simulink model "LB_PathTracAdptVel_EKF"  (Simulink 9.2)
settings: Solver=ode4  StartTime=0  StopTime=400  FixedStep=1e-3  RelTol=1e-6  AbsTol=1e-6
InitFcn:
  | clear;
  | close all
StopFcn:
  | close all;
  | t=tout(1:length(Vel_Trg));
  | figure
  | subplot(2,1,1)
  | plot(PreView_X,PreView_Y,'r','LineWidth',1.5);
  | hold on
  | plot(Current_Position(:,1),Current_Position(:,2),'k','LineWidth',1.5);
  | legend('Preview Position','Current Position');
  | 
  | subplot(2,1,2)
  | plot(Cur_Yaw,'r','LineWidth',1.5);
  | hold on
  | plot(PreViewHeading,'k','LineWidth',1.5);
  | legend('Current Heading','PreView Heading');
  | 
  | figure
  | subplot(3,1,1)
  | plot(Delta_Lateral,'k','LineWidth',1.5);
  | legend('Lateral Errors');
  | subplot(3,1,2)
  | plot(Heading_error,'r','LineWidth',1.5);
  | legend('Heading  Errors');
  | subplot(3,1,3)
  | plot(SteerCmd,'k','LineWidth',1.5);
  | legend('Steering Command');
  | 
  | % figure
  | % subplot(2,1,1)
  | % plot(ax_Cur,'k','LineWidth',1.5);
  | % legend('Longitudinal Acceleration')
  | % hold on
  | % subplot(2,1,2)
  | % plot(ay_Cur,'r','LineWidth',1.5);
  | % legend('Lateral Acceleration')
  | 
  | %% 加噪后的测量vs真实值
  | figure1=figure;
  | axes1 = axes('Parent',figure1);
  | hold(axes1,'on');
  | plot(Xo_Ce,Yo_Ce,'b','LineWidth',1)
  | hold on
  | plot(Xo_Cur,Yo_Cur,'-.r','LineWidth',2)
  | legend('测量值','真实值')
  | % 创建 ylabel
  | ylabel({'Y-m'});
  | xlabel({'X-m'});
  | box(axes1,'on');
  | grid(axes1,'on');
  | % 设置其余坐标区属性
  | set(axes1,'FontName','Times New Roman','FontWeight','bold');
  | 
  | 
  | figure2=figure;
  | axes2 = axes('Parent',figure2);
  | hold(axes2,'on');
  | plot(t,ax_Ce,'b','LineWidth',1)
  | hold on
  | plot(t,ax_Cur,'-.r','LineWidth',2)
  | legend('测量值','真实值')
  | % 创建 ylabel
  | ylabel({'纵向加速度-m/s^2'});
  | xlabel({'时间-s'});
  | box(axes2,'on');
  | grid(axes2,'on');
  | % 设置其余坐标区属性
  | set(axes2,'FontName','Times New Roman','FontWeight','bold');
  | 
  | figure4=figure;
  | axes4 = axes('Parent',figure4);
  | hold(axes4,'on');
  | plot(t,ay_Ce,'b','LineWidth',1)
  | hold on
  | plot(t,ay_Cur,'-.r','LineWidth',2)
  | legend('测量值','真实值')
  | % 创建 ylabel
  | ylabel({'横向加速度-m/s^2'});
  | xlabel({'时间-s'});
  | box(axes4,'on');
  | grid(axes4,'on');
  | % 设置其余坐标区属性
  | set(axes4,'FontName','Times New Roman','FontWeight','bold');
  | 
  | figure3=figure;
  | axes3 = axes('Parent',figure3);
  | hold(axes3,'on');
  | plot(t,Yaw_Ce,'b','LineWidth',1)
  | hold on
  | plot(t,Yaw_Cur,'-.r','LineWidth',2)
  | legend('测量值','真实值')
  | % 创建 ylabel
  | ylabel({'横摆角-rad'});
  | xlabel({'时间-s'});
  | box(axes3,'on');
  | grid(axes3,'on');
  | % 设置其余坐标区属性
  | set(axes3,'FontName','Times New Roman','FontWeight','bold');
  | %% EKF 结果图
  | figure_Position=figure;
  | axes4 = axes('Parent',figure_Position);
  | hold(axes4,'on');
  | plot(X_Groud_Truth(:,1),X_Groud_Truth(:,2),'r','LineWidth',2)
  | hold on
  | % plot(tout,Yaw,'-.r','LineWidth',2)
  | plot(X_EKF_Opt(:,1),X_EKF_Opt(:,2),'b','LineWidth',2)
  | plot(X_Ce_Current(:,1),X_Ce_Current(:,2),'k','LineWidth',2)
  | legend('真实值','EKF-估计','测量值')
  | % 创建 ylabel
  | ylabel({'Y-m'});
  | xlabel({'X-m'});
  | box(axes4,'on');
  | grid(axes4,'on');
  | % 设置其余坐标区属性
  | set(axes4,'FontName','Times New Roman','FontWeight','bold');
  | 
  | figure_Yaw=figure;
  | axes5 = axes('Parent',figure_Yaw);
  | hold(axes5,'on');
  | plot(t,X_Groud_Truth(:,3),'r','LineWidth',2)
  | hold on
  | plot(t,X_EKF_Opt(:,3),'b','LineWidth',2)
  | plot(t,X_Ce_Current(:,3),'k','LineWidth',2)
  | legend('真实值','EKF-估计','测量值')
  | % 创建 ylabel
  | ylabel({'航向角-rad'});
  | xlabel({'时间-s'});
  | box(axes5,'on');
  | grid(axes5,'on');
  | % 设置其余坐标区属性
  | set(axes5,'FontName','Times New Roman','FontWeight','bold');
  | 
  | figure_YawRate=figure;
  | axes6 = axes('Parent',figure_YawRate);
  | hold(axes6,'on');
  | plot(t,X_Groud_Truth(:,4),'r','LineWidth',2)
  | hold on
  | plot(t,X_EKF_Opt(:,4),'b','LineWidth',2)
  | plot(t,X_Ce_Current(:,4),'k','LineWidth',2)
  | legend('真实值','EKF-估计','测量值')
  | % 创建 ylabel
  | ylabel({'横摆角速度-rad/s'});
  | xlabel({'时间-s'});
  | box(axes6,'on');
  | grid(axes6,'on');
  | % 设置其余坐标区属性
  | set(axes6,'FontName','Times New Roman','FontWeight','bold');
  | 
  | figure_Vx=figure;
  | axes7 = axes('Parent',figure_Vx);
  | hold(axes7,'on');
  | plot(t,X_Groud_Truth(:,5),'r','LineWidth',2)
  | hold on
  | plot(t,X_EKF_Opt(:,5),'b','LineWidth',2)
  | % plot(t,X_Ce_Current(:,4),'k','LineWidth',2)
  | legend('真实值','EKF-估计')
  | % 创建 ylabel
  | ylabel({'纵向车速-m/s'});
  | xlabel({'时间-s'});
  | box(axes7,'on');
  | grid(axes7,'on');
  | % 设置其余坐标区属性
  | set(axes7,'FontName','Times New Roman','FontWeight','bold');
  | 
  | figure_Vy=figure;
  | axes8 = axes('Parent',figure_Vy);
  | hold(axes8,'on');
  | plot(t,X_Groud_Truth(:,6),'r','LineWidth',2)
  | hold on
  | plot(t,X_EKF_Opt(:,6),'b','LineWidth',2)
  | % plot(t,X_Ce_Current(:,4),'k','LineWidth',2)
  | legend('真实值','EKF-估计')
  | % 创建 ylabel
  | ylabel({'横向车速-m/s'});
  | xlabel({'时间-s'});
  | box(axes8,'on');
  | grid(axes8,'on');
  | % 设置其余坐标区属性
  | set(axes8,'FontName','Times New Roman','FontWeight','bold');
libraries: simulink x9, Solver_SF x1
settings Model: Creator=ywata  LastModifiedBy=Administrator  SimulationMode=accelerator  ExtModeTrigMode=oneshot  ExtModeArmWhenConnect=off
settings SolverCC: AutoScaleAbsTol=off
settings DataIOCC: LimitDataPoints=off  SignalLoggingName=sigsOut
settings OptimizationCC: BlockReduction=off  BooleanDataType=off
settings DebuggingCC: SaveWithParameterizedLinksMsg=none  SignalResolutionControl=TryResolveAllWithWarning  MultiTaskDSMMsg=warning  MultiTaskCondExecSysMsg=none
settings HardwareCC: TargetUnknown=on
settings RTWCC: TemplateMakefile=grt_vc.tmf
settings GRTTargetCC: TargetFcnLib=ansi_tfl_tmw.mat

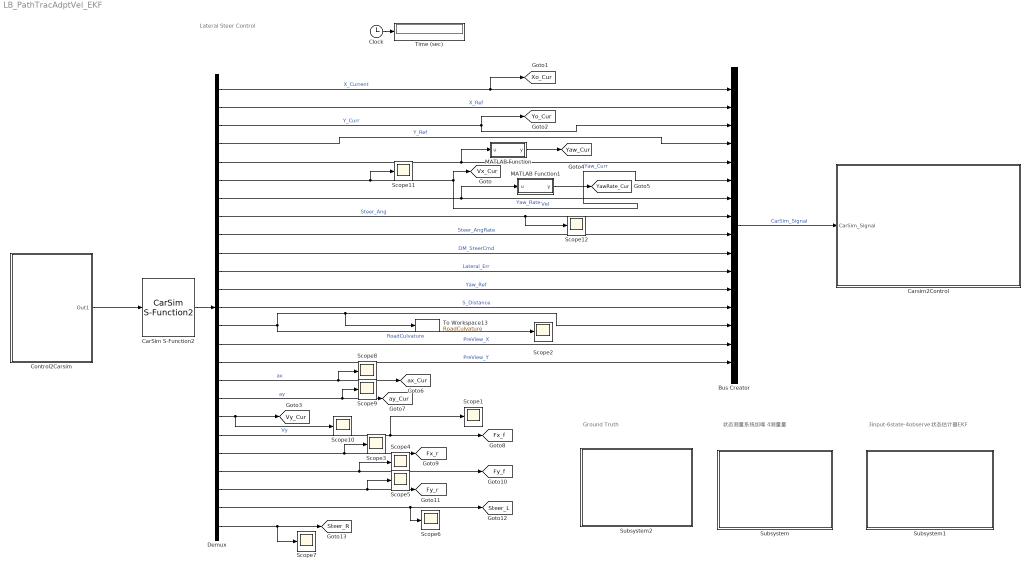
== system LB_PathTracAdptVel_EKF ==
  note: Lateral Steer Control
  note: 状态测量系统加噪
      | 4测量量
  note: 3input-6state-4observe状态估计器EKF
  note: Ground Truth
  Bus Creator : BusCreator  Inputs=16
  CarSim S-Function2 : Solver_SF/CarSim S-Function2  Priority=1  VehicleCode=i_i  SIMFILE=simfile.sim
      settings: AttributesFormatString=Vehicle Code: %<VehicleCode>
  Carsim2Control : Subsystem
  Clock : Clock
  Control2Carsim : Subsystem
  Demux : Demux  Outputs=25
  MATLAB Function : MATLAB Function  TreatAsAtomicUnit=on
  MATLAB Function1 : MATLAB Function  TreatAsAtomicUnit=on
  Scope{1..12} (12 alike) : Scope
  Subsystem : Subsystem
  Subsystem1 : Subsystem
  Subsystem2 : Subsystem
  Time (sec) : Display
      settings: Format=bank  Decimation=100
  To Workspace13 : ToWorkspace  VariableName=RoadCulvature  SampleTime=-1
  tag scope: Fx_f=global, Fx_r=global, Fy_f=global, Fy_r=global, Steer_L=global, Steer_R=global, Vx_Cur=global, Vy_Cur=global, Xo_Cur=global, YawRate_Cur=global, Yaw_Cur=global, Yo_Cur=global, ax_Cur=global, ay_Cur=global
  wires:
  CarSim S-Function2/1 -> Demux/1
  Clock/1 -> Time (sec)/1
  Demux/1 -> [Xo_Cur], Bus Creator/1  "X_Current"
  Demux/2 -> Bus Creator/2  "X_Ref"
  Demux/3 -> [Yo_Cur], Bus Creator/3  "Y_Curr"
  Demux/4 -> Bus Creator/4  "Y_Ref"
  Demux/5 -> MATLAB Function/1(u), Bus Creator/5  "Yaw_Curr"
  Demux/6 -> Scope11/1, [Vx_Cur], Bus Creator/6  "Vel"
  Demux/8 -> Scope12/1, Bus Creator/8  "Steer_Ang"
  Demux/9 -> Bus Creator/9  "Steer_AngRate"
  Demux/10 -> Bus Creator/10  "DM_SteerCmd"
  Demux/11 -> Bus Creator/11  "Lateral_Err"
  Demux/12 -> Bus Creator/12  "Yaw_Ref"
  Demux/13 -> Bus Creator/13  "S_Distance"
  Demux/14 -> Scope2/1, To Workspace13/1, Bus Creator/14  "RoadCulvature"
  Demux/15 -> Bus Creator/15  "PreView_X"
  Demux/16 -> Bus Creator/16  "PreView_Y"
  Bus Creator/1 -> Carsim2Control/1(CarSim_Signal)  "CarSim_Signal"
  Control2Carsim/1(Out1) -> CarSim S-Function2/1
  Demux/18 -> Scope9/1, [ay_Cur]  "ay"
  Demux/17 -> Scope8/1, [ax_Cur]  "ax"
  MATLAB Function1/1(y) -> [YawRate_Cur]
  Demux/7 -> MATLAB Function1/1(u), Bus Creator/7  "Yaw_Rate"
  MATLAB Function/1(y) -> [Yaw_Cur]
  Demux/19 -> Scope10/1, [Vy_Cur]  "Vy"
  Demux/20 -> Scope1/1, [Fx_f]
  Demux/21 -> Scope3/1, [Fx_r]
  Demux/22 -> Scope4/1, [Fy_f]
  Demux/23 -> Scope5/1, [Fy_r]
  Demux/24 -> Scope6/1, [Steer_L]
  Demux/25 -> Scope7/1, [Steer_R]

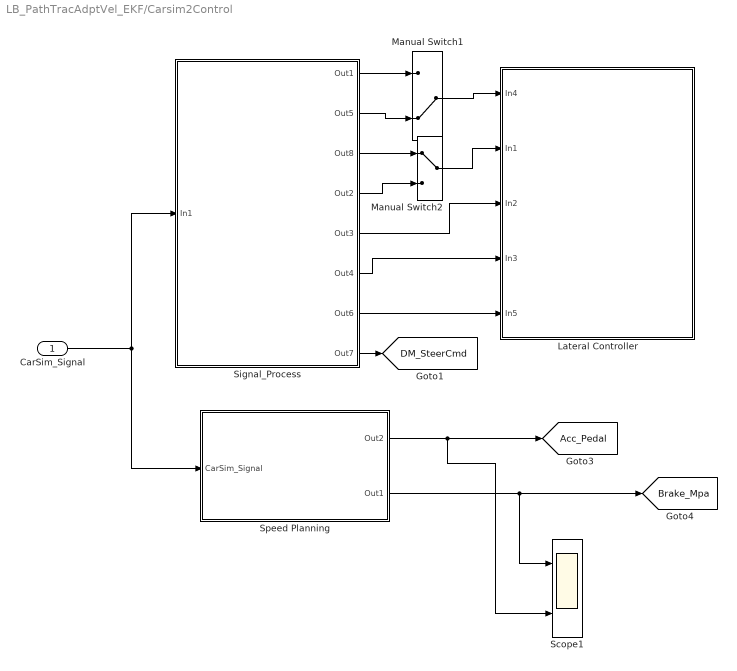
== system LB_PathTracAdptVel_EKF/Carsim2Control ==
  CarSim_Signal : Inport
  Lateral Controller : Subsystem
  Manual Switch1 : ManualSwitch  CurrentSetting=0
  Manual Switch2 : ManualSwitch
  Scope1 : Scope  NumInputPorts=2
  "Signal_Process " : Subsystem
  Speed Planning : Subsystem
  tag scope: Acc_Pedal=global, Brake_Mpa=global, DM_SteerCmd=global
  wires:
  "Signal_Process "/7(Out6) -> Lateral Controller/5(In5)
  Manual Switch1/1 -> Lateral Controller/1(In4)
  CarSim_Signal/1 -> Speed Planning/1(CarSim_Signal), "Signal_Process "/1(In1)
  "Signal_Process "/4(Out2) -> Manual Switch2/2
  Manual Switch2/1 -> Lateral Controller/2(In1)
  "Signal_Process "/2(Out5) -> Manual Switch1/2
  "Signal_Process "/8(Out7) -> [DM_SteerCmd]
  Speed Planning/1(Out2) -> Scope1/2, [Acc_Pedal]
  "Signal_Process "/3(Out8) -> Manual Switch2/1
  Speed Planning/2(Out1) -> Scope1/1, [Brake_Mpa]
  "Signal_Process "/1(Out1) -> Manual Switch1/1
  "Signal_Process "/5(Out3) -> Lateral Controller/3(In2)
  "Signal_Process "/6(Out4) -> Lateral Controller/4(In3)

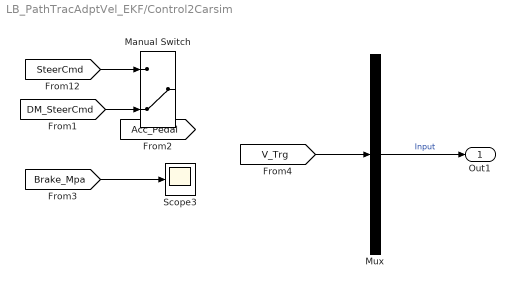
== system LB_PathTracAdptVel_EKF/Control2Carsim ==
  Manual Switch : ManualSwitch  CurrentSetting=0
  Mux : Mux  Inputs=1
  Scope3 : Scope
  Out1 : Outport
  wires:
  [SteerCmd] -> Manual Switch/1
  Mux/1 -> Out1/1  "Input"
  [DM_SteerCmd] -> Manual Switch/2
  [Brake_Mpa] -> Scope3/1
  [V_Trg] -> Mux/1

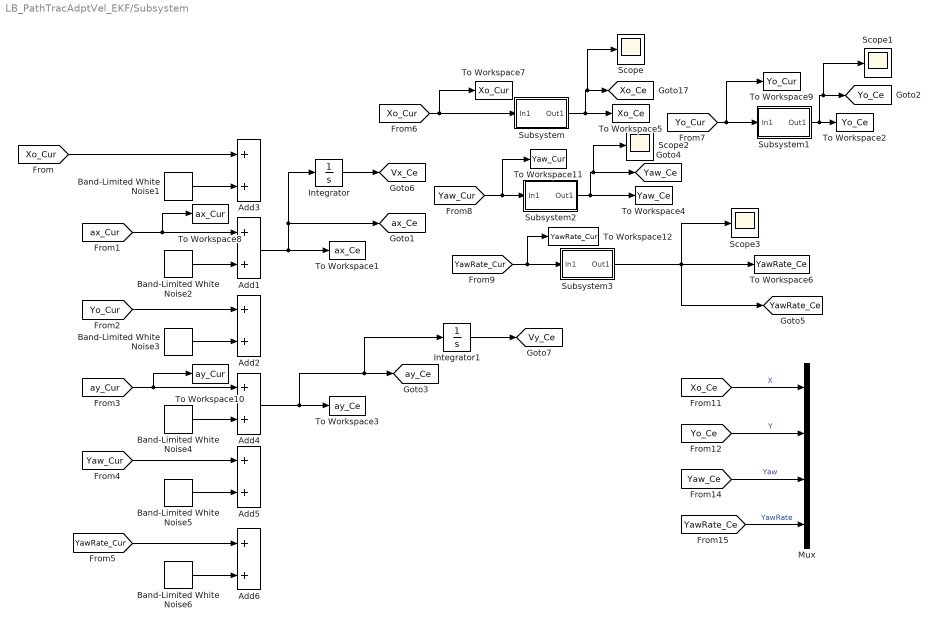
== system LB_PathTracAdptVel_EKF/Subsystem ==
  Add{1..6} (6 alike) : Sum
  Band-Limited White Noise1 : simulink/Sources/Band-Limited White Noise  Cov=0.0001*[0.1]  Ts=1e-3  seed=[23341]
  Band-Limited White Noise2 : simulink/Sources/Band-Limited White Noise  Cov=0.001*[0.1]  Ts=1e-3  seed=[23341]
  Band-Limited White Noise3 : simulink/Sources/Band-Limited White Noise  Cov=0.0001*[0.1]  Ts=1e-3  seed=[23341]
  Band-Limited White Noise4 : simulink/Sources/Band-Limited White Noise  Cov=0.001*[0.1]  Ts=1e-3  seed=[23341]
  Band-Limited White Noise5 : simulink/Sources/Band-Limited White Noise  Cov=0.000003*[0.1]  Ts=1e-3  seed=[23341]
  Band-Limited White Noise6 : simulink/Sources/Band-Limited White Noise  Cov=0.00003*[0.1]  Ts=1e-3  seed=[23341]
  Integrator : Integrator
  Integrator1 : Integrator
  Mux : Mux
  Scope{,1..3} (4 alike) : Scope
  Subsystem : Subsystem  mask{Delta=0.1}
      mask prompts: Delta "标准差"
  Subsystem1 : Subsystem  mask{Delta=0.1}
      mask prompts: Delta "标准差"
  Subsystem2 : Subsystem  mask{Delta=deg2rad(3)}
      mask prompts: Delta "标准差"
  Subsystem3 : Subsystem  mask{Delta=deg2rad(1)}
      mask prompts: Delta "标准差"
  To Workspace1 : ToWorkspace  VariableName=ax_Ce  SampleTime=-1
  To Workspace10 : ToWorkspace  VariableName=ay_Cur  SampleTime=-1
  To Workspace11 : ToWorkspace  VariableName=Yaw_Cur  SampleTime=-1
  To Workspace12 : ToWorkspace  VariableName=YawRate_Cur  SampleTime=-1
  To Workspace2 : ToWorkspace  VariableName=Yo_Ce  SampleTime=-1
  To Workspace3 : ToWorkspace  VariableName=ay_Ce  SampleTime=-1
  To Workspace4 : ToWorkspace  VariableName=Yaw_Ce  SampleTime=-1
  To Workspace5 : ToWorkspace  VariableName=Xo_Ce  SampleTime=-1
  To Workspace6 : ToWorkspace  VariableName=YawRate_Ce  SampleTime=-1
  To Workspace7 : ToWorkspace  VariableName=Xo_Cur  SampleTime=-1
  To Workspace8 : ToWorkspace  VariableName=ax_Cur  SampleTime=-1
  To Workspace9 : ToWorkspace  VariableName=Yo_Cur  SampleTime=-1
  tag scope: Vx_Ce=global, Vy_Ce=global, Xo_Ce=global, YawRate_Ce=global, Yaw_Ce=global, Yo_Ce=global, ax_Ce=global, ay_Ce=global
  wires:
  Band-Limited White Noise1/1 -> Add3/2
  [Xo_Cur] -> Add3/1
  [ax_Cur] -> To Workspace8/1, Add1/1
  Band-Limited White Noise2/1 -> Add1/2
  Band-Limited White Noise3/1 -> Add2/2
  [Yo_Cur] -> Add2/1
  [ay_Cur] -> To Workspace10/1, Add4/1
  Band-Limited White Noise4/1 -> Add4/2
  Add4/1 -> Integrator1/1, [ay_Ce], To Workspace3/1
  Band-Limited White Noise5/1 -> Add5/2
  [Yaw_Cur] -> Add5/1
  [YawRate_Cur] -> Add6/1
  Band-Limited White Noise6/1 -> Add6/2
  Add1/1 -> [ax_Ce], Integrator/1, To Workspace1/1
  Integrator/1 -> [Vx_Ce]
  Integrator1/1 -> [Vy_Ce]
  [Yaw_Ce] -> Mux/3  "Yaw"
  [YawRate_Ce] -> Mux/4  "YawRate"
  [Xo_Ce] -> Mux/1  "X"
  [Yo_Ce] -> Mux/2  "Y"
  Subsystem/1(Out1) -> Scope/1, [Xo_Ce], To Workspace5/1
  [Xo_Cur] -> To Workspace7/1, Subsystem/1(In1)
  [Yo_Cur] -> To Workspace9/1, Subsystem1/1(In1)
  Subsystem1/1(Out1) -> Scope1/1, [Yo_Ce], To Workspace2/1
  Subsystem2/1(Out1) -> To Workspace4/1, Scope2/1, [Yaw_Ce]
  [Yaw_Cur] -> To Workspace11/1, Subsystem2/1(In1)
  [YawRate_Cur] -> To Workspace12/1, Subsystem3/1(In1)
  Subsystem3/1(Out1) -> To Workspace6/1, Scope3/1, [YawRate_Ce]

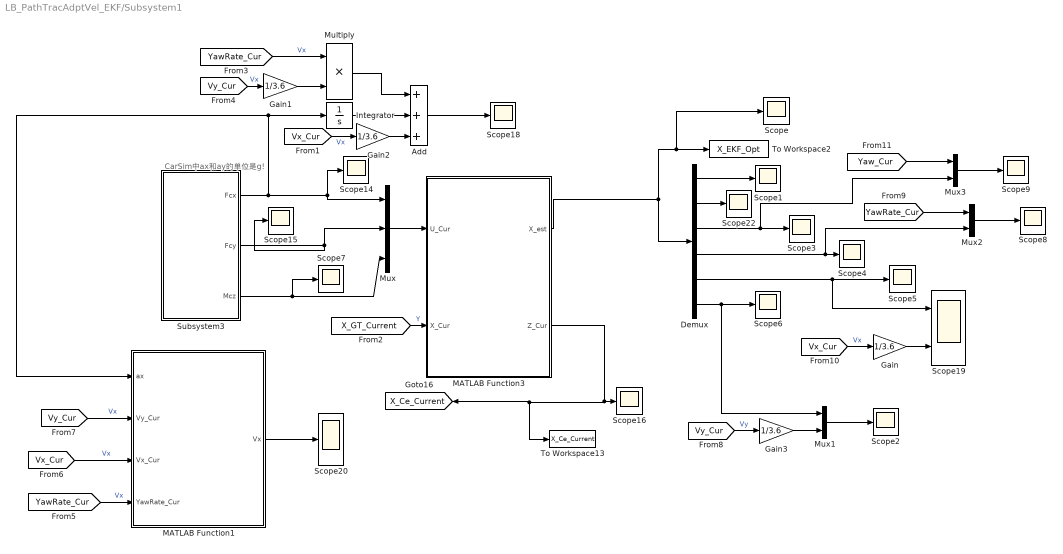
== system LB_PathTracAdptVel_EKF/Subsystem1 ==
  note: CarSim中ax和ay的单位是g!
  Add : Sum  Inputs=+++
  Demux : Demux  Outputs=6
  Gain{,1..3} (4 alike) : Gain  Gain=1/3.6
  Integrator : Integrator
  MATLAB Function1 : MATLAB Function  TreatAsAtomicUnit=on
  MATLAB Function3 : MATLAB Function  TreatAsAtomicUnit=on
  Multiply : Product
  Mux : Mux  Inputs=3
  Mux1 : Mux  Inputs=2
  Mux2 : Mux  Inputs=2
  Mux3 : Mux  Inputs=2
  Scope{,1..9,14..16,18,20,22} (16 alike) : Scope
  Scope19 : Scope  NumInputPorts=2
  Subsystem3 : Subsystem
  To Workspace13 : ToWorkspace  VariableName=X_Ce_Current  SampleTime=-1
      settings: Save2DSignal=2-D array (concatenate along first dimension)
  To Workspace2 : ToWorkspace  VariableName=X_EKF_Opt  SampleTime=-1
      settings: Save2DSignal=2-D array (concatenate along first dimension)
  tag scope: X_Ce_Current=global
  wires:
  [X_GT_Current] -> MATLAB Function3/2(X_Cur)  "Y"
  Demux/1 -> Scope1/1
  Demux/2 -> Scope22/1
  Demux/5 -> Scope19/1, Scope5/1
  Demux/6 -> Mux1/1, Scope6/1
  MATLAB Function3/1(X_est) -> Demux/1, Scope/1, To Workspace2/1
  MATLAB Function3/2(Z_Cur) -> To Workspace13/1, [X_Ce_Current], Scope16/1
  Mux/1 -> MATLAB Function3/1(U_Cur)
  Integrator/1 -> Add/2
  [Vx_Cur] -> Gain/1  "Vx"
  Gain/1 -> Scope19/2
  [Vx_Cur] -> Gain2/1  "Vx"
  Add/1 -> Scope18/1
  [YawRate_Cur] -> Multiply/1  "Vx"
  Gain1/1 -> Multiply/2
  [Vy_Cur] -> Gain1/1  "Vx"
  Multiply/1 -> Add/1
  Gain2/1 -> Add/3
  [YawRate_Cur] -> MATLAB Function1/4(YawRate_Cur)  "Vx"
  [Vx_Cur] -> MATLAB Function1/3(Vx_Cur)  "Vx"
  [Vy_Cur] -> MATLAB Function1/2(Vy_Cur)  "Vx"
  MATLAB Function1/1(Vx) -> Scope20/1
  Subsystem3/1(Fcx) -> Scope14/1, Mux/1, Integrator/1, MATLAB Function1/1(ax)
  Subsystem3/2(Fcy) -> Mux/2, Scope15/1
  Subsystem3/3(Mcz) -> Mux/3, Scope7/1
  [Vy_Cur] -> Gain3/1  "Vy"
  Gain3/1 -> Mux1/2
  Mux1/1 -> Scope2/1
  Mux2/1 -> Scope8/1
  Demux/4 -> Mux2/2, Scope4/1
  [YawRate_Cur] -> Mux2/1
  [Yaw_Cur] -> Mux3/1
  Demux/3 -> Mux3/2, Scope3/1
  Mux3/1 -> Scope9/1

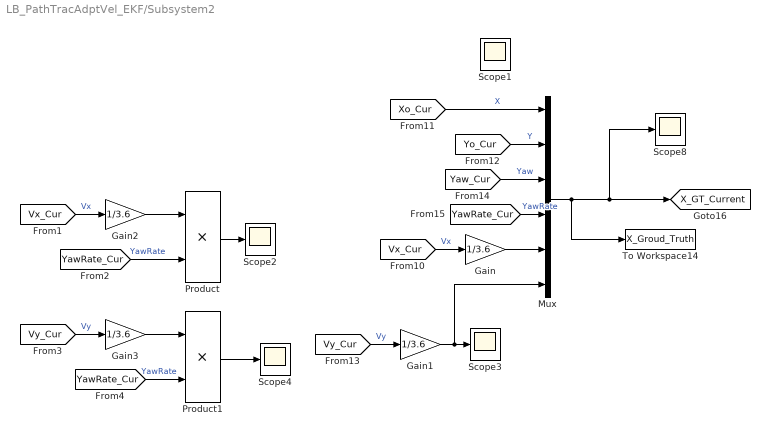
== system LB_PathTracAdptVel_EKF/Subsystem2 ==
  Gain{,1..3} (4 alike) : Gain  Gain=1/3.6
  Mux : Mux  Inputs=6
  Product : Product
  Product1 : Product
  Scope{1..4,8} (5 alike) : Scope
  To Workspace14 : ToWorkspace  VariableName=X_Groud_Truth  SampleTime=-1
      settings: Save2DSignal=2-D array (concatenate along first dimension)
  tag scope: X_GT_Current=global
  wires:
  [Xo_Cur] -> Mux/1  "X"
  Mux/1 -> To Workspace14/1, Scope8/1, [X_GT_Current]
  [Vy_Cur] -> Gain1/1  "Vy"
  [Vx_Cur] -> Gain/1  "Vx"
  Gain1/1 -> Mux/6, Scope3/1
  [Vx_Cur] -> Gain2/1  "Vx"
  Gain2/1 -> Product/1
  [YawRate_Cur] -> Product/2  "YawRate"
  Product/1 -> Scope2/1
  [Vy_Cur] -> Gain3/1  "Vy"
  Gain3/1 -> Product1/1
  [YawRate_Cur] -> Product1/2  "YawRate"
  Product1/1 -> Scope4/1
  [Yo_Cur] -> Mux/2  "Y"
  [Yaw_Cur] -> Mux/3  "Yaw"
  [YawRate_Cur] -> Mux/4  "YawRate"
  Gain/1 -> Mux/5

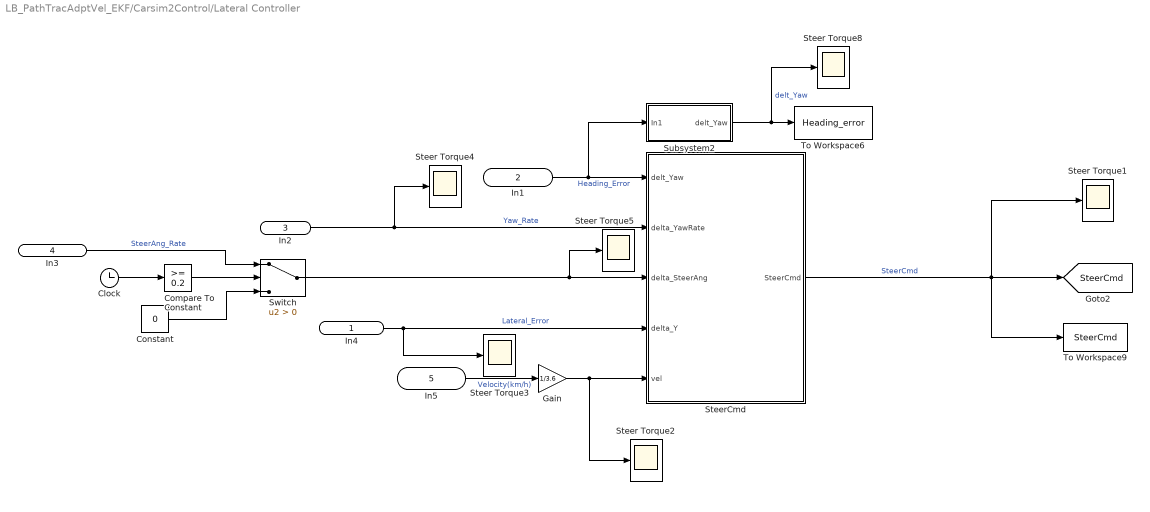
== system LB_PathTracAdptVel_EKF/Carsim2Control/Lateral Controller ==
  In4 : Inport
  In1 : Inport  Port=2
  In2 : Inport  Port=3
  In3 : Inport  Port=4
  In5 : Inport  Port=5
  Clock : Clock
  Compare To Constant : simulink/Logic and Bit Operations/Compare To Constant  relop=>=  const=0.2  OutDataTypeStr=boolean
  Constant : Constant  Value=0
  Gain : Gain  Gain=1/3.6
  Steer Torque{1..5,8} (6 alike) : Scope
  SteerCmd : MATLAB Function  TreatAsAtomicUnit=on
  Subsystem2 : Subsystem
  Switch : Switch  Criteria=u2 > Threshold
  To Workspace6 : ToWorkspace  VariableName=Heading_error  SampleTime=-1
  To Workspace9 : ToWorkspace  VariableName=SteerCmd  SampleTime=-1
  tag scope: SteerCmd=global
  wires:
  In5/1 -> Gain/1  "Velocity(km/h)"
  SteerCmd/1(SteerCmd) -> [SteerCmd], Steer Torque1/1, To Workspace9/1  "SteerCmd"
  Gain/1 -> Steer Torque2/1, SteerCmd/5(vel)
  In2/1 -> Steer Torque4/1, SteerCmd/2(delta_YawRate)  "Yaw_Rate"
  In1/1 -> Subsystem2/1(In1), SteerCmd/1(delt_Yaw)  "Heading_Error"
  In4/1 -> Steer Torque3/1, SteerCmd/4(delta_Y)  "Lateral_Error"
  Subsystem2/1(delt_Yaw) -> Steer Torque8/1, To Workspace6/1  "delt_Yaw"
  Clock/1 -> Compare To Constant/1
  Compare To Constant/1 -> Switch/2
  In3/1 -> Switch/1  "SteerAng_Rate"
  Constant/1 -> Switch/3
  Switch/1 -> Steer Torque5/1, SteerCmd/3(delta_SteerAng)

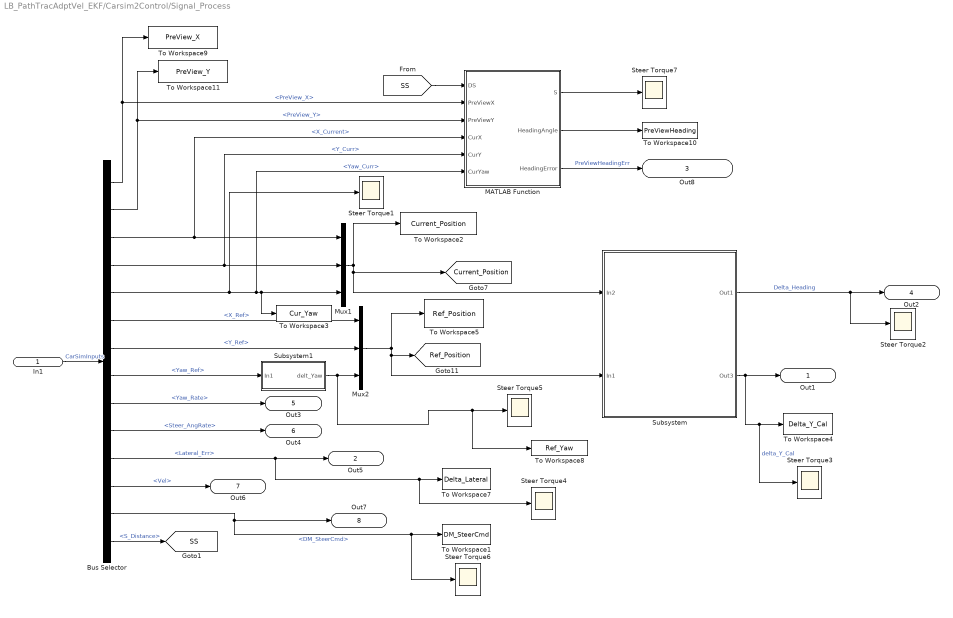
== system LB_PathTracAdptVel_EKF/Carsim2Control/Signal_Process  ==
  In1 : Inport
  Bus Selector : BusSelector  OutputSignals=PreView_X,PreView_Y,X_Current,Y_Curr,Yaw_Curr,X_Ref,Y_Ref,Yaw_Ref,Yaw_Rate,Steer_AngRate,Lateral_Err,Vel,DM_SteerCmd,S_Distance
  MATLAB Function : MATLAB Function  TreatAsAtomicUnit=on
  Mux1 : Mux  Inputs=3
  Mux2 : Mux  Inputs=3
  Steer Torque{1..7} (7 alike) : Scope
  Subsystem : Subsystem
  Subsystem1 : Subsystem
  To Workspace1 : ToWorkspace  VariableName=DM_SteerCmd  SampleTime=-1
  To Workspace10 : ToWorkspace  VariableName=PreViewHeading  SampleTime=-1
  To Workspace11 : ToWorkspace  VariableName=PreView_Y  SampleTime=-1
  To Workspace2 : ToWorkspace  VariableName=Current_Position  SampleTime=-1
  To Workspace3 : ToWorkspace  VariableName=Cur_Yaw  SampleTime=-1
  To Workspace4 : ToWorkspace  VariableName=Delta_Y_Cal  SampleTime=-1
  To Workspace5 : ToWorkspace  VariableName=Ref_Position  SampleTime=-1
  To Workspace7 : ToWorkspace  VariableName=Delta_Lateral  SampleTime=-1
  To Workspace8 : ToWorkspace  VariableName=Ref_Yaw  SampleTime=-1
  To Workspace9 : ToWorkspace  VariableName=PreView_X  SampleTime=-1
  Out1 : Outport
  Out5 : Outport  Port=2
  Out8 : Outport  Port=3
  Out2 : Outport  Port=4
  Out3 : Outport  Port=5
  Out4 : Outport  Port=6
  Out6 : Outport  Port=7
  Out7 : Outport  Port=8
  tag scope: Current_Position=global, Ref_Position=global, SS=global
  wires:
  Mux1/1 -> Subsystem/1(In2), [Current_Position], To Workspace2/1
  Bus Selector/6 -> Mux2/1  "<X_Ref>"
  Bus Selector/7 -> Mux2/2  "<Y_Ref>"
  Mux2/1 -> Subsystem/2(In1), [Ref_Position], To Workspace5/1
  Subsystem/1(Out1) -> Steer Torque2/1, Out2/1  "Delta_Heading"
  In1/1 -> Bus Selector/1  "CarSimInputs"
  Bus Selector/3 -> MATLAB Function/4(CurX), Mux1/1  "<X_Current>"
  Bus Selector/4 -> MATLAB Function/5(CurY), Mux1/2  "<Y_Curr>"
  Bus Selector/5 -> Steer Torque1/1, Mux1/3, To Workspace3/1, MATLAB Function/6(CurYaw)  "<Yaw_Curr>"
  Bus Selector/8 -> Subsystem1/1(In1)  "<Yaw_Ref>"
  Subsystem1/1(delt_Yaw) -> To Workspace8/1, Steer Torque5/1, Mux2/3
  Subsystem/2(Out3) -> Steer Torque3/1, To Workspace4/1, Out1/1  "delta_Y_Cal"
  Bus Selector/10 -> Out4/1  "<Steer_AngRate>"
  Bus Selector/9 -> Out3/1  "<Yaw_Rate>"
  Bus Selector/11 -> Steer Torque4/1, To Workspace7/1, Out5/1  "<Lateral_Err>"
  Bus Selector/12 -> Out6/1  "<Vel>"
  Bus Selector/13 -> Out7/1, Steer Torque6/1, To Workspace1/1  "<DM_SteerCmd>"
  Bus Selector/14 -> [SS]  "<S_Distance>"
  MATLAB Function/3(HeadingError) -> Out8/1  "PreViewHeadingErr"
  MATLAB Function/2(HeadingAngle) -> To Workspace10/1
  Bus Selector/1 -> To Workspace9/1, MATLAB Function/2(PreViewX)  "<PreView_X>"
  Bus Selector/2 -> To Workspace11/1, MATLAB Function/3(PreViewY)  "<PreView_Y>"
  MATLAB Function/1(S) -> Steer Torque7/1
  [SS] -> MATLAB Function/1(DS)

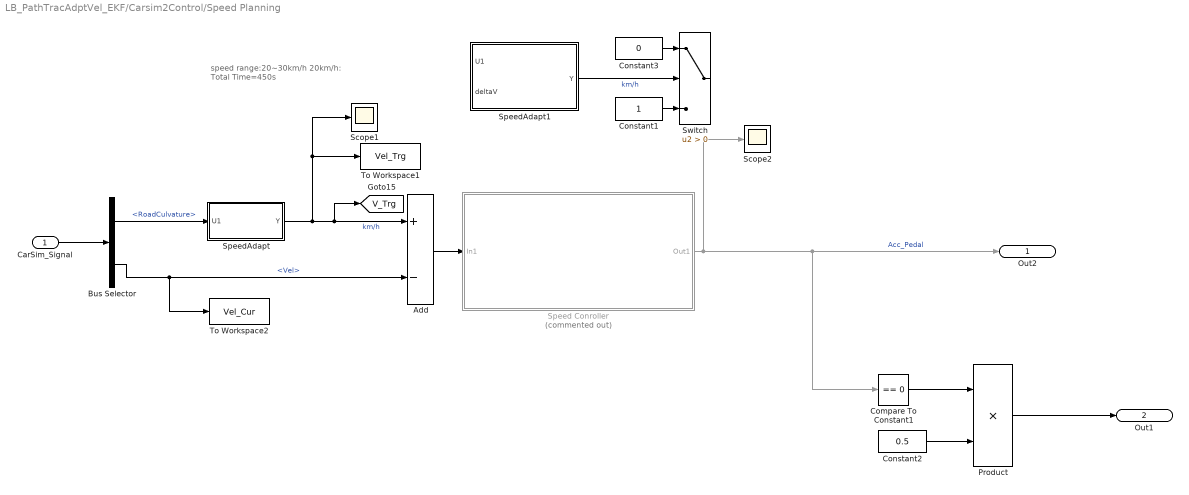
== system LB_PathTracAdptVel_EKF/Carsim2Control/Speed Planning ==
  note: speed range:20~30km/h
      | 20km/h: Total Time=450s
  CarSim_Signal : Inport
  Add : Sum  Inputs=+-
  Bus Selector : BusSelector  OutputSignals=RoadCulvature,Vel
  Compare To Constant1 : simulink/Logic and Bit Operations/Compare To Constant  relop===  const=0  OutDataTypeStr=boolean
  Constant1 : Constant
  Constant2 : Constant  Value=0.5
  Constant3 : Constant  Value=0
  Product : Product
  Scope1 : Scope
  Scope2 : Scope
  Speed Conroller : Subsystem  Commented=on
  SpeedAdapt : MATLAB Function  TreatAsAtomicUnit=on
  SpeedAdapt1 : MATLAB Function  TreatAsAtomicUnit=on
  Switch : Switch  Criteria=u2 > Threshold
  To Workspace1 : ToWorkspace  VariableName=Vel_Trg  SampleTime=-1
      settings: Save2DSignal=2-D array (concatenate along first dimension)
  To Workspace2 : ToWorkspace  VariableName=Vel_Cur  SampleTime=-1
      settings: Save2DSignal=2-D array (concatenate along first dimension)
  Out2 : Outport
  Out1 : Outport  Port=2
  tag scope: V_Trg=global
  wires:
  Add/1 -> Speed Conroller/1(In1)
  CarSim_Signal/1 -> Bus Selector/1
  Bus Selector/2 -> To Workspace2/1, Add/2  "<Vel>"
  Bus Selector/1 -> SpeedAdapt/1(U1)  "<RoadCulvature>"
  SpeedAdapt/1(Y) -> To Workspace1/1, Scope1/1, [V_Trg], Add/1  "km/h"
  Constant2/1 -> Product/2
  Speed Conroller/1(Out1) -> Out2/1, Compare To Constant1/1, Scope2/1  "Acc_Pedal"
  Constant1/1 -> Switch/3
  Constant3/1 -> Switch/1
  SpeedAdapt1/1(Y) -> Switch/2  "km/h"
  Compare To Constant1/1 -> Product/1
  Product/1 -> Out1/1

== system LB_PathTracAdptVel_EKF/Subsystem/Subsystem ==
  In1 : Inport
  Constant : Constant  Value=Delta
  MATLAB Function : MATLAB Function  TreatAsAtomicUnit=on
  Out1 : Outport
  wires:
  Constant/1 -> MATLAB Function/1(delta)
  In1/1 -> MATLAB Function/2(u)
  MATLAB Function/1(y) -> Out1/1

== system LB_PathTracAdptVel_EKF/Subsystem/Subsystem1 ==
  In1 : Inport
  Constant : Constant  Value=Delta
  MATLAB Function : MATLAB Function  TreatAsAtomicUnit=on
  Out1 : Outport
  wires:
  MATLAB Function/1(y) -> Out1/1
  In1/1 -> MATLAB Function/2(u)
  Constant/1 -> MATLAB Function/1(delta)

== system LB_PathTracAdptVel_EKF/Subsystem/Subsystem2 ==
  In1 : Inport
  Constant : Constant  Value=Delta
  MATLAB Function : MATLAB Function  TreatAsAtomicUnit=on
  Out1 : Outport
  wires:
  Constant/1 -> MATLAB Function/1(delta)
  In1/1 -> MATLAB Function/2(u)
  MATLAB Function/1(y) -> Out1/1

== system LB_PathTracAdptVel_EKF/Subsystem/Subsystem3 ==
  In1 : Inport
  Constant : Constant  Value=Delta
  MATLAB Function : MATLAB Function  TreatAsAtomicUnit=on
  Out1 : Outport
  wires:
  MATLAB Function/1(y) -> Out1/1
  In1/1 -> MATLAB Function/2(u)
  Constant/1 -> MATLAB Function/1(delta)

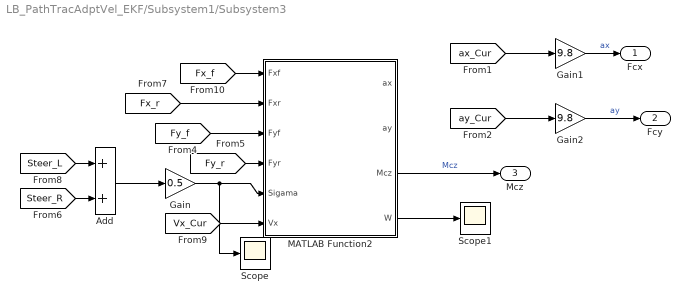
== system LB_PathTracAdptVel_EKF/Subsystem1/Subsystem3 ==
  Add : Sum
  Gain : Gain  Gain=0.5
  Gain1 : Gain  Gain=9.8
  Gain2 : Gain  Gain=9.8
  MATLAB Function2 : MATLAB Function  TreatAsAtomicUnit=on
  Scope : Scope
  Scope1 : Scope
  Fcx : Outport
  Fcy : Outport  Port=2
  Mcz : Outport  Port=3
  wires:
  [Fy_r] -> MATLAB Function2/4(Fyr)
  [Vx_Cur] -> MATLAB Function2/6(Vx)
  [Fy_f] -> MATLAB Function2/3(Fyf)
  MATLAB Function2/3(Mcz) -> Mcz/1  "Mcz"
  [ay_Cur] -> Gain2/1
  [ax_Cur] -> Gain1/1
  [Steer_L] -> Add/1
  [Steer_R] -> Add/2
  Add/1 -> Gain/1
  Gain/1 -> Scope/1, MATLAB Function2/5(Sigama)
  [Fx_r] -> MATLAB Function2/2(Fxr)
  [Fx_f] -> MATLAB Function2/1(Fxf)
  Gain1/1 -> Fcx/1  "ax"
  Gain2/1 -> Fcy/1  "ay"
  MATLAB Function2/4(W) -> Scope1/1

== system LB_PathTracAdptVel_EKF/Carsim2Control/Lateral Controller/Subsystem2 ==
  In1 : Inport
  Rad2Deg1 : MATLAB Function  TreatAsAtomicUnit=on
  delt_Yaw : Outport
  wires:
  Rad2Deg1/1(Y) -> delt_Yaw/1  "Deg"
  In1/1 -> Rad2Deg1/1(U1)  "rad"

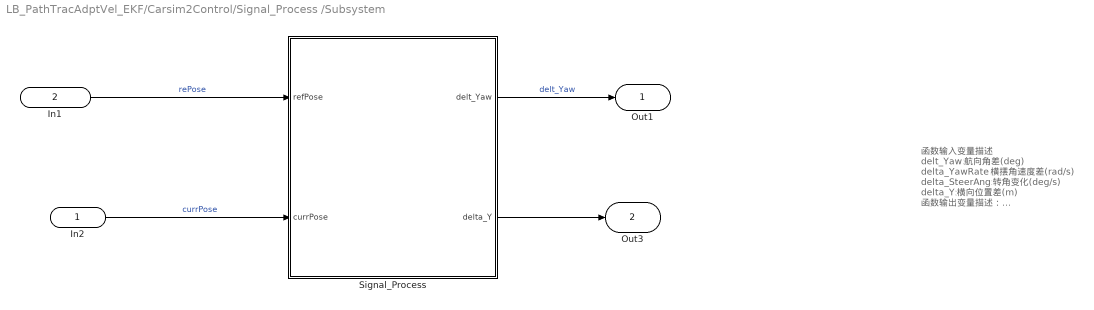
== system LB_PathTracAdptVel_EKF/Carsim2Control/Signal_Process /Subsystem ==
  note: 函数输入变量描述
      | delt_Yaw:航向角差(deg)
      | delta_YawRate:横摆角速度差(rad/s)
      | delta_SteerAng:转角变化(deg/s)
      | delta_Y:横向位置差(m)
      | 函数输出变量描述：
      | SteerCmd:前轮转角（degree）
  In2 : Inport
  In1 : Inport  Port=2
  Signal_Process : MATLAB Function  TreatAsAtomicUnit=on
  Out1 : Outport
  Out3 : Outport  Port=2
  wires:
  In1/1 -> Signal_Process/1(refPose)  "rePose"
  Signal_Process/1(delt_Yaw) -> Out1/1  "delt_Yaw"
  In2/1 -> Signal_Process/2(currPose)  "currPose"
  Signal_Process/2(delta_Y) -> Out3/1

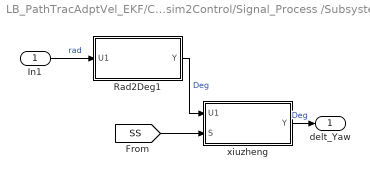
== system LB_PathTracAdptVel_EKF/Carsim2Control/Signal_Process /Subsystem1 ==
  In1 : Inport
  Rad2Deg1 : MATLAB Function  TreatAsAtomicUnit=on
  xiuzheng : MATLAB Function  TreatAsAtomicUnit=on
  delt_Yaw : Outport
  wires:
  In1/1 -> Rad2Deg1/1(U1)  "rad"
  Rad2Deg1/1(Y) -> xiuzheng/1(U1)  "Deg"
  [SS] -> xiuzheng/2(S)
  xiuzheng/1(Y) -> delt_Yaw/1  "Deg"

== system LB_PathTracAdptVel_EKF/Carsim2Control/Speed Planning/Speed Conroller ==
  In1 : Inport
  Constant : Constant  Value=0.2
  Constant1 : Constant  Value=0.1
  Discrete Varying PID : simulink/Continuous/PID Controller  Controller=PI  Form=Parallel  TimeDomain=Discrete-time  SampleTime=-1  IntegratorMethod=Forward Euler  FilterMethod=Forward Euler  ControllerParametersSource=external  P=1  I=1  D=0  UseFilter=on  N=100  TunerSelectOption=Transfer Function Based (PID Tuner App)  InitialConditionSource=internal  InitialConditionForIntegrator=0  InitialConditionForFilter=0  DifferentiatorICPrevScaledInput=0  ExternalReset=none  TrackingMode=off  Kt=1  LimitOutput=on  UpperSaturationLimit=1  LowerSaturationLimit=0  LinearizeAsGain=on  AntiWindupMode=none  Kb=1  POutMin=[]  POutMax=[]  IOutMin=[]  IOutMax=[]  DOutMin=[]  DOutMax=[]  NOutMin=[]  NOutMax=[]  SumOutMin=[]  SumOutMax=[]  SaturationOutMin=[]  SaturationOutMax=[]  PParamMin=[]  PParamMax=[]  IParamMin=[]  IParamMax=[]  DParamMin=[]  DParamMax=[]  NParamMin=[]  NParamMax=[]  KbParamMin=[]  KbParamMax=[]  KtParamMin=[]  KtParamMax=[]  KbOutMin=[]  KbOutMax=[]  KtOutMin=[]  KtOutMax=[]  IntegratorOutMin=[]  IntegratorOutMax=[]  FilterOutMin=[]  FilterOutMax=[]  SumI1OutMin=[]  SumI1OutMax=[]  SumI2OutMin=[]  SumI2OutMax=[]  SumI3OutMin=[]  SumI3OutMax=[]  SumI4OutMin=[]  SumI4OutMax=[]  SumDOutMin=[]  SumDOutMax=[]  DifferentiatorOutMin=[]  DifferentiatorOutMax=[]  FilterDiffOutCoefMin=[]  FilterDiffOutCoefMax=[]  ReciprocalOutMin=[]  ReciprocalOutMax=[]  SumDenOutMin=[]  SumDenOutMax=[]  SumNumOutMin=[]  SumNumOutMax=[]  DivideOutMin=[]  DivideOutMax=[]  IntegratorContinuousStateAttributes=''  IntegratorStateMustResolveToSignalObject=off  IntegratorRTWStateStorageClass=Auto  FilterContinuousStateAttributes=''  FilterStateMustResolveToSignalObject=off  FilterRTWStateStorageClass=Auto  ParallelPVariant=ExternalParameters  IdealPVariant=Disabled  IVariant=ExternalParameters  DVariant=Disabled  IntegratorVariant=Discrete  SatVariant=Enabled  AWVariant=Passthrough  PCopyVariant=Disabled  TRVariant=Disabled  FdbkBlocksVariant=Forward  IdealPFdbkVariant=Disabled  SatFdbkVariant=Disabled  DerivativeFilterVariant=Disabled  NVariant=Disabled  NCopyVariant=Disabled_SignalSpec  FilterICVariant=Disabled  IntegratorICVariant=InternalICs  ExternalResetVariant=Disabled  TRSumVariant=Passthrough  SumFdbkVariant=Disabled  SumVariant=Sum_PI
  Out1 : Outport
  wires:
  Constant/1 -> Discrete Varying PID/3
  In1/1 -> Discrete Varying PID/1  "Error_Spd"
  Constant1/1 -> Discrete Varying PID/2
  Discrete Varying PID/1 -> Out1/1  "Acc_Pedal"

== matlab function Carsim2Control/Signal_Process /Subsystem/Signal_Process ==
  data: refPose input double; delt_Yaw output double; currPose input double; delta_Y output double
function [delt_Yaw,delta_Y] = Signal_Process(refPose, currPose)
 % Clip heading angle to be within [0, 360) and convert to radian
refPose(3) = matlabshared.planning.internal.angleUtilities.convertAndWrapTo2Pi(refPose(3));
currPose(3)= matlabshared.planning.internal.angleUtilities.convertAndWrapTo2Pi(currPose(3));
delt_Yaw=matlabshared.planning.internal.angleUtilities.angdiff(refPose(3), currPose(3));
direction=1;
wheelbase=3;
delta_Y = computePositionError(refPose, currPose, direction, wheelbase);
end

 function delta_Y = computePositionError(refPose, currPose, direction, wheelbase)
% %computePositionError Compute the distance error
% 
% Tangent direction of the reference path
tHat = [cos(refPose(3)), sin(refPose(3))];

% Tracking error vector
if 1
    [poseF1,poseF2] = rearToFrontPose(currPose, wheelbase);
    d1 = poseF1 - refPose(1);
    d2 = poseF2 - refPose(2);

else
    d1 = currPose(1)  - refPose(1);
    d2 = currPose(2)  - refPose(2);
end
% 
% % Implement equation (8) in reference [2]
delta_Y = -(d1*tHat(2) - d2*tHat(1));

 end

  function [poseF1,poseF2]  = rearToFrontPose(currPose, wheelbase)
%rearPoseToFrontPose Transform pose from rear wheel to front wheel

% %   Copyright 2018 The MathWorks, Inc.
% 
% %#internal
% %#codegen
poseF1=currPose(1);
poseF2=currPose(2);
poseF1 = poseF1 + wheelbase * cos(currPose(3));
poseF2 = poseF2 + wheelbase * sin(currPose(3));

end

== matlab function Carsim2Control/Lateral Controller/Subsystem2/Rad2Deg1 ==
  data: U1 input double; Y output double
function Y= Signal_Process(U1)
Y=rad2deg(U1);
end

== matlab function Carsim2Control/Lateral Controller/SteerCmd ==
  data: delt_Yaw input double; SteerCmd output double; delta_YawRate input double; delta_SteerAng input double; delta_Y input double; vel input double
function SteerCmd = Signal_Process(delt_Yaw,delta_YawRate, delta_SteerAng, ...
    delta_Y,vel)
k1=10;
k2=1;
k3=1;
k4=1;
% delt_Yaw=deg2rad(delt_Yaw);
SteerCmd=-3*(delt_Yaw+atan(k1*delta_Y/(k2+vel)-0.85*deg2rad(delta_SteerAng))-(delta_YawRate~=0)*(vel/200*delta_YawRate));% 前轮转角 
maxSteer=540;
% Saturate and convert to degree
SteerCmd = saturate(rad2deg(SteerCmd), maxSteer);

end

%--------------------------------------------------------------------------
%--------------------------------------------------------------------------
% Helper function
%--------------------------------------------------------------------------
%--------------------------------------------------------------------------
function delta = saturate(delta, maxSteeringAngle)
%saturate Saturate steering angle when it exceeds MaxSteeringAngle
delta = sign(delta) * min(abs(delta), maxSteeringAngle);
end

== matlab function Carsim2Control/Signal_Process /Subsystem1/xiuzheng ==
  data: U1 input double; Y output double; S input double
function Y= Signal_Process(U1,S)
if U1>=0||S>1000
    Y=U1-359.785;
else
    Y=U1;
end
end

== matlab function Carsim2Control/Signal_Process /Subsystem1/Rad2Deg1 ==
  data: U1 input double; Y output double
function Y= Signal_Process(U1)
Y=rad2deg(U1);
end

== matlab function Carsim2Control/Speed Planning/SpeedAdapt ==
  data: U1 input double; Y output double
function Y= SpeedAdaptive(U1)
Y=30-8*abs(U1*100)/4;
Y = round(Y);
end

== matlab function Carsim2Control/Speed Planning/SpeedAdapt1 ==
  data: U1 input double; Y output double; deltaV input double
function Y= BrakeInterval(U1,deltaV)
if U1<=0.1&&deltaV<0
    Y=1;
else
    Y=0;
end
end

== matlab function Carsim2Control/Signal_Process /MATLAB Function ==
  data: DS input double; PreViewX input double; PreViewY input double; CurX input double; S output double; HeadingAngle output double; CurY input double; HeadingError output double; CurYaw input double
function [S,HeadingAngle,HeadingError] = fcn(DS,PreViewX,PreViewY,CurX,CurY,CurYaw)
C1=0;
deltaX=PreViewX-CurX;
deltaY=PreViewY-CurY;
S=norm([deltaX deltaY]);
C1=rad2deg(atan2(deltaY,deltaX));%-pi到pi之间的值
HeadingAngle1 = matlabshared.planning.internal.angleUtilities.convertAndWrapTo2Pi(C1);
CurYaw= matlabshared.planning.internal.angleUtilities.convertAndWrapTo2Pi(CurYaw);
HeadingError=matlabshared.planning.internal.angleUtilities.angdiff(HeadingAngle1, CurYaw);
if DS>1000||C1>0
HeadingAngle=C1-359.785;
else
HeadingAngle=C1;
end
end

== matlab function MATLAB Function1 ==
  data: u input double; y output double
function y = fcn(u)

y = deg2rad(u);

== matlab function MATLAB Function ==
  data: u input double; y output double
function y = fcn(u)

y = deg2rad(u);

== matlab function Subsystem/Subsystem/MATLAB Function ==
  data: delta input double; u input double; y output double
function y = fcn(delta,u)
%#codegen

y = u+delta*randn;

== matlab function Subsystem1/MATLAB Function3 ==
  settings: updateMethod=DISCRETE
  data: U_Cur input double; X_est output double; X_Cur input double; Z_Cur output double
function [X_est,Z_Cur] = fcn(U_Cur,X_Cur)
persistent X_est_1 Pk 
if isempty(X_est_1)
    X_est_1 = X_Cur;
    %% 误差协方差矩阵
Pk = 0.1*eye(6);
    %% 误差协方差矩阵

end

%% 常数设置
Ts = 1e-3;%跟仿真步长设置有关
Iz = 1343;%转动惯量
%% 系统误差向量
q = [2e-1 2e-1 1e-6 5e-1 1e-5 1e-5 ];
% q = zeros(1,6);
%% 测量误差向量
r = [0.2 0.2 0.00349 0.00349];
%% 输入
u1 = U_Cur(1);
u2 = U_Cur(2);
u3 = U_Cur(3)/Iz;
%% 测量加噪
Z_C1= X_Cur(1)+r(1)*(1-2*rand);
Z_C2= X_Cur(2)+r(2)*(1-2*rand);
Z_C3= X_Cur(3)+r(3)*(1-2*rand);
Z_C4= X_Cur(4)+r(4)*(1-2*rand);

Z_Cur =[Z_C1 Z_C2 Z_C3 Z_C4]';
%% 上一步最有估计状态
x1 = X_est_1(1);
x2 = X_est_1(2);
x3 = X_est_1(3);
x4 = X_est_1(4);
x5 = X_est_1(5);
x6 = X_est_1(6);

%% 噪声矩阵
Qk = diag(q)^2;
Rk = diag(r)^2;
%% 当前测量
% Z_Cur = Z_Ce_Curr;
%% 状态转移矩阵 
Ad=[1 0 -Ts*x5*sin(x3)-Ts*x6*cos(x3) 0 Ts*cos(x3) -Ts*sin(x3);
    0 1 Ts*x5*cos(x3)-Ts*x6*sin(x3) 0 Ts*sin(x3) Ts*cos(x3);
    0 0 1 Ts 0 0;
    0 0 0 1 0 0;
    0 0 0 Ts*x6 1 Ts*x4;
    0 0 0 -Ts*x5 -Ts*x4 1];
%% 观测矩阵
Cd=[1 0 0 0 0 0;
    0 1 0 0 0 0;
    0 0 1 0 0 0;
    0 0 0 1 0 0];
%% 模型估计值
x1_next = Ts*(x5*cos(x3)-x6*sin(x3))+x1;
x2_next = Ts*(x5*sin(x3)+x6*cos(x3))+x2;
x3_next = Ts*x4 + x3;
x4_next = Ts*u3 + x4;
x5_next = Ts*u1 +Ts*x4*x6 + x5;
x6_next = Ts*u2 - Ts*x4*x5 + x6;
x_forecast = [x1_next x2_next x3_next x4_next x5_next x6_next]';

%%
% Vx1 = Vx1+(U_Cur(1)+X_est_1(4)*X_est_1(6))*Ts;
% 
% Vx2 = Vx2+(U_Cur(1)+X_Cur_1(4)*X_Cur_1(6))*Ts;
% 
% Vx = Vx1 + X_est_1(2);
% 
% Vxx = Vx2+X_Cur_1(2);

%% 测量预测
z1 = x1_next;
z2 = x2_next;
z3 = x3_next;
z4 = x4_next;
Z_yuce = [z1 z2 z3 z4]';
%% 误差协方差矩阵预更新
Pkk_1 = Ad*Pk*Ad'+Ts^2*Qk;
%% 卡尔曼增益计算
%  Kk = Pkk_1*Cd'*(Cd*Pkk_1*Cd'+Rk)^-1;       %计算增益
 Kk = Pkk_1*Cd'*inv(Cd*Pkk_1*Cd'+Rk);       %计算增益
%% 最优估计
 x_hat = x_forecast+Kk*(Z_Cur-Z_yuce);      %校正
 %% 更新协方差矩阵
 Pk = (eye(6)-Kk*Cd)*Pkk_1;
 X_est = x_hat;
 X_est_1 = X_est;

== matlab function Subsystem/Subsystem1/MATLAB Function ==
  data: delta input double; u input double; y output double
function y = fcn(delta,u)
%#codegen

y = u+delta*randn;

== matlab function Subsystem1/Subsystem3/MATLAB Function2 ==
  data: Fxf input double; Fxr input double; ax output double; Fyf input double; Fyr input double; Sigama input double; Vx input double; ay output double; Mcz output double; W output double
function [ax,ay,Mcz,W] = fcn(Fxf,Fxr,Fyf,Fyr,Sigama,Vx)
% coder.extrinsic('dsearchn'); 
Fx = Fxf+Fxr;
Lf=1.04;
Lr=1.56;
Cd=0.28;
A=2.8;
m = 1110;
Sigama=deg2rad(Sigama);
Fcx=Fx*cos(Sigama)-Fyr*sin(Sigama)-Cd*A*Vx^2/21.15;
Fcy = Fx*sin(Sigama)+Fyf*cos(Sigama)+Fyr;

Mcz=Fyf*Lf*cos(Sigama)+Fxf*Lf*sin(Sigama)-Fyr*Lr;

% Mcz=Fyf*Lf*cos(Sigama)+Fx*Lf*sin(Sigama)-Fyr*Lr;
ax = Fcx/m;
ay = Fcy/m;
W = Mcz/1200;

== matlab function Subsystem/Subsystem2/MATLAB Function ==
  data: delta input double; u input double; y output double
function y = fcn(delta,u)
%#codegen

y = u+delta*randn;

== matlab function Subsystem/Subsystem3/MATLAB Function ==
  data: delta input double; u input double; y output double
function y = fcn(delta,u)
%#codegen

y = u+delta*randn;

== matlab function Subsystem1/MATLAB Function1 ==
  data: ax input double; Vy_Cur input double; Vx output double; Vx_Cur input double; YawRate_Cur input double
function Vx  = fcn(ax,Vy_Cur,Vx_Cur,YawRate_Cur)
persistent Vx1 Vx2
Ts = 1e-4;
if isempty(Vx1)
    Vx1 = 0;
end
if isempty(Vx2)
    Vx2 = 0;
end
Vx1 = Vx1+ax*Ts;
Vx2 = Vx2+(ax+Vy_Cur*YawRate_Cur/3.6)*Ts;

Vx = Vx2+Vx_Cur/3.6;
